simulink model "TCSILOW"  (R2019a)
settings: Solver=VariableStepAuto  StartTime=0.0  StopTime=100  FixedStep=0.001  RelTol=1e-5  AbsTol=1e-5  EnableMultiTasking=on
values from neighbouring files (symbols this model uses):
  beta0 = 47.9602    [Model_Parameter_TCSI_A.m]
  beta2 = 2.1291e-005    (= 2.1291e-05)    [Model_Parameter_TCSI_A.m]
  BSR_opt = 0.9755    [Model_Parameter_TCSI_A.m]
  c_mlin = 1.4021    [Model_Parameter_TCSI_A.m]
  c_mVec = [1.3563 2.7692e+03 0.0100]    [Model_Parameter_TCSI_A.m]
  c_pa = 1011    [Model_Parameter_TCSI_A.m]
  c_pe = 1332    [Model_Parameter_TCSI_A.m]
  c_phi2 = 0    [Model_Parameter_TCSI_A.m]
  c_pi = 0.2708    [Model_Parameter_TCSI_A.m]
  c_psi2 = 0    [Model_Parameter_TCSI_A.m]
  c_wphiVec = [-1.4298e-08 -0.0015 29.6462]    [Model_Parameter_TCSI_A.m]
  c_wpsiVec = [1.0882e-08 -1.7320e-04 1.0286]    [Model_Parameter_TCSI_A.m]
  d_th = 32e-3    (= 0.032)    [Model_Parameter_TCSI_A.m]
  eta0 = 0.41512    [Model_Parameter_TCSI_A.m]
  eta1 = 6.9379e-005    (= 6.9379e-05)    [Model_Parameter_TCSI_A.m]
  eta_cmax = 0.7364    [Model_Parameter_TCSI_A.m]
  eta_tmmax = 0.8180    (= 0.818)    [Model_Parameter_TCSI_A.m]
  gamma0 = 0.5337    [Model_Parameter_TCSI_A.m]
  gamma1 = 4e-3    (= 0.004)    [Model_Parameter_TCSI_A.m]
  gamma2 = -9.4152e-6    (= -9.4152e-06)    [Model_Parameter_TCSI_A.m]
  gamma_a = 1.3964    [Model_Parameter_TCSI_A.m]
  gamma_e = 1.2734    [Model_Parameter_TCSI_A.m]
  I_e = 0.32074    [Model_Parameter_TCSI_A.m]
  J_t = 2.0000e-04    (= 0.0002)    [Model_Parameter_TCSI_A.m]
  kappa = 1.35    [Model_Parameter_TCSI_A.m]
  lambda = 1    [Model_Parameter_TCSI_A.m]
  LHV = 42.5e6    (= 42500000)    [Model_Parameter_TCSI_A.m]
  p_a = 0.98e5    (= 98000)    [Model_Parameter_TCSI_A.m]
  p_e = 1.05e5    (= 105000)    [Model_Parameter_TCSI_A.m]
  p_minit = 3e4    (= 30000)    [Model_Parameter_TCSI_A.m]
  pi_copt = 1.0455    [Model_Parameter_TCSI_A.m]
  Q_c = [3.09189776853185,-2.48232013831700;-2.48232013831700,2.14785596204381]    [Model_Parameter_TCSI_A.m]
  R = 287    [Model_Parameter_TCSI_A.m]
  R_a = 287    [Model_Parameter_TCSI_A.m]
  R_c = 0.0400    (= 0.04)    [Model_Parameter_TCSI_A.m]
  R_t = 0.0400    (= 0.04)    [Model_Parameter_TCSI_A.m]
  sigma_0 = 14.7    [Model_Parameter_TCSI_A.m]
  theta_a = 298    [Model_Parameter_TCSI_A.m]
  theta_exm = 873    [Model_Parameter_TCSI_A.m]
  theta_m = 298    [Model_Parameter_TCSI_A.m]
  u_0 = 0.0039    [Model_Parameter_TCSI_A.m]
  V_c = 1.99e-3    (= 0.00199)    [Model_Parameter_TCSI_A.m]
  V_d = 0.0127    [Model_Parameter_TCSI_A.m]
  V_exm = 0.0012    [Model_Parameter_TCSI_A.m]
  V_m = 16.3210e-3    (= 0.016321)    [Model_Parameter_TCSI_A.m]
  w_copt = 0.2753    [Model_Parameter_TCSI_A.m]
  w_tlin = 2.7969e+03    (= 2796.9)    [Model_Parameter_TCSI_A.m]
undefined symbols (not defined in the file or in its folder): den, num
libraries: simulink x10, cstblocks x1
settings Model: Creator=GOBA  LastModifiedBy=ameya
settings SolverCC: ZeroCrossAlgorithm=Adaptive
settings DataIOCC: ExternalInput=[0 2]  InitialState=[]  LimitDataPoints=on  LoadInitialState=on  SaveFormat=Array  SignalLoggingSaveFormat=ModelDataLogs  ReturnWorkspaceOutputs=off  SignalLoggingName=sigsOut
settings OptimizationCC: DefaultParameterBehavior=Inlined  BufferReuse=off  ExpressionDepthLimit=2147483647  InitFltsAndDblsToZero=on  LifeSpan=inf
settings DebuggingCC: SaveWithParameterizedLinksMsg=none  UnderspecifiedInitializationDetection=Classic  MergeDetectMultiDrivingBlocksExec=none  SignalResolutionControl=TryResolveAllWithWarning  IgnoredZcDiagnostic=none  MultiTaskDSMMsg=warning  MultiTaskCondExecSysMsg=none  FcnCallInpInsideContextMsg=warning  StateNameClashWarn=warning  InitInArrayFormatMsg=none  SFUnexpectedBacktrackingDiag=warning  SFNoUnconditionalDefaultTransitionDiag=warning  SFExecutionAtInitializationDiag=none  ArithmeticOperatorsInVariantConditions=warning
settings HardwareCC: ProdBitPerPointer=32  ProdBitPerSizeT=32  ProdBitPerPtrDiffT=32  ProdLargestAtomicFloat=None  ProdIntDivRoundTo=Undefined  ProdEndianess=Unspecified  ProdWordSize=32  ProdHWDeviceType=32-bit Generic  TargetUnknown=on
settings ModelReferenceCC: PropagateSignalLabelsOutOfModel=off
settings SFSimCC: SimUseLocalCustomCode=off
settings RTWCC: Description=Generic Real-Time Target  RTWUseLocalCustomCode=off
settings CodeAppCC: StateflowObjectComments=on
settings GRTTargetCC: TargetFcnLib=ansi_tfl_tmw.mat  TargetLangStandard=C89/C90 (ANSI)  GeneratePreprocessorConditionals=Disable all  CombineOutputUpdateFcns=off  GRTInterface=on
settings ConfigComp: CovMetricSettings=dw  CovHtmlReporting=on  CovSaveCumulativeToWorkspaceVar=on  CovSaveSingleToWorkspaceVar=on  CovExternalEMLEnable=off

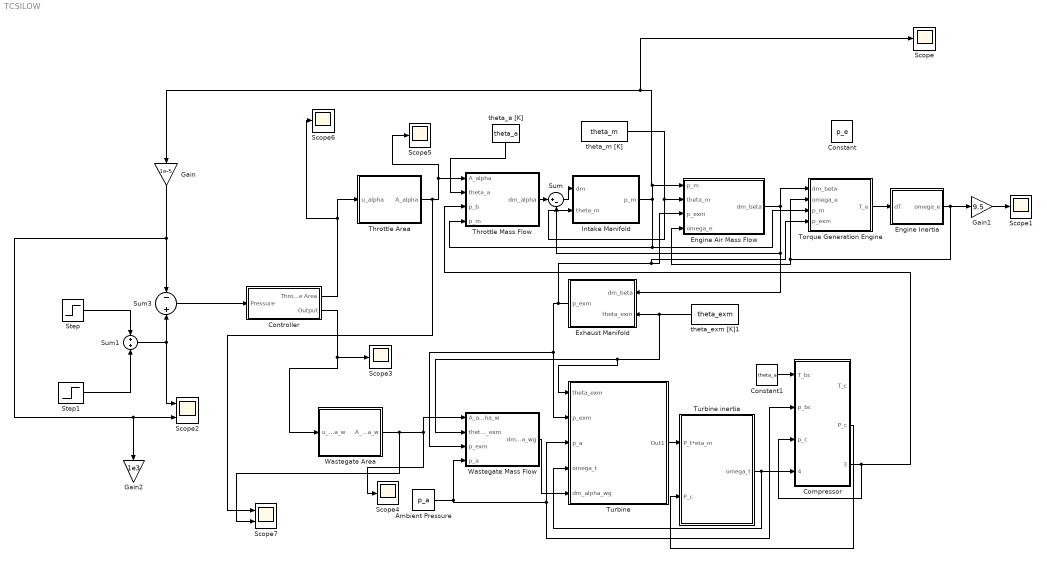
== system TCSILOW ==
  Ambient Pressure : Constant  Value=p_a
  "Compressor " : Subsystem
  Constant : Constant  Value=p_e
  Constant1 : Constant  Value=theta_a
  Controller : Subsystem
  Engine Air Mass Flow : Subsystem
  Engine Inertia : Subsystem
  Exhaust Manifold : Subsystem
  Gain : Gain  Gain=1e-5
  Gain1 : Gain  Gain=9.5
  Gain2 : Gain  Gain=1e3
  Intake Manifold : Subsystem
  Scope{,1,3..6} (6 alike) : Scope
  Scope2 : Scope  NumInputPorts=2
  Scope7 : Scope  NumInputPorts=2
  Step : Step  Time=20  Before=0.3  After=0.6  SampleTime=0
  Step1 : Step  Time=65  After=0.3  SampleTime=0
  Sum : Sum  Inputs=|+-  SaturateOnIntegerOverflow=on
  Sum1 : Sum
  Sum3 : Sum  Inputs=-+
  Throttle Area : Subsystem
  Throttle Mass Flow : Subsystem
  Torque Generation Engine : Subsystem
  "Turbine " : Subsystem
  "Turbine inertia " : Subsystem
  Wastegate Area : Subsystem
  Wastegate Mass Flow : Subsystem
  theta_a [K] : Constant  Value=theta_a
  theta_exm [K]1 : Constant  Value=theta_exm
  theta_m [K] : Constant  Value=theta_m
  wires:
  theta_a [K]/1 -> Throttle Mass Flow/2(theta_a)
  Throttle Mass Flow/1(dm_alpha) -> Sum/1
  Sum/1 -> Intake Manifold/1(dm)
  Torque Generation Engine/1(T_e) -> Engine Inertia/1(dT)
  theta_exm [K]1/1 -> "Turbine "/1(theta_exm), Wastegate Mass Flow/2(theta_exm), Exhaust Manifold/2(theta_exm)
  Exhaust Manifold/1("p_exm ") -> Torque Generation Engine/4(p_exm), Engine Air Mass Flow/3(p_exm), "Turbine "/2(p_exm), Wastegate Mass Flow/3(p_exm)
  Engine Air Mass Flow/1(dm_beta) -> Torque Generation Engine/1(dm_beta), Exhaust Manifold/1(dm_beta), Sum/2
  Wastegate Mass Flow/1(dm_alpha_wg) -> "Turbine "/5(dm_alpha_wg)
  Controller/1(Throttle Area) -> Scope6/1, Throttle Area/1(u_alpha)
  Engine Inertia/1("omega_e ") -> Engine Air Mass Flow/4(omega_e), Torque Generation Engine/2(omega_e), Gain1/1
  Ambient Pressure/1 -> "Compressor "/2(p_bc), "Turbine "/3(p_a), Wastegate Mass Flow/4(p_a)
  Controller/2(Output) -> Scope3/1, Wastegate Area/1(u_alpha_w)
  "Turbine "/1(Out1) -> "Turbine inertia "/1(P_t*eta_m)
  "Turbine inertia "/1(omega_t) -> "Turbine "/4(omega_t), "Compressor "/4(omega_t1)
  "Compressor "/2(P_c) -> "Turbine inertia "/2(P_c)
  "Compressor "/3(p_boost) -> "Compressor "/3(p_c), Throttle Mass Flow/3(p_b)
  Constant1/1 -> "Compressor "/1(T_bc)
  Gain1/1 -> Scope1/1
  Wastegate Area/1(A_alpha_w) -> Scope7/2, Wastegate Mass Flow/1(A_alpha_w), Scope4/1
  Intake Manifold/1("p_m ") -> Torque Generation Engine/3(p_m), Throttle Mass Flow/4(p_m), Engine Air Mass Flow/1(p_m), Scope/1, Gain/1
  Sum3/1 -> Controller/1(Pressure)
  Gain/1 -> Scope2/2, Gain2/1, Sum3/1
  theta_m [K]/1 -> Intake Manifold/2(theta_m), Engine Air Mass Flow/2(theta_m)
  Step/1 -> Sum1/1
  Step1/1 -> Sum1/2
  Sum1/1 -> Sum3/2, Scope2/1
  Throttle Area/1(A_alpha) -> Throttle Mass Flow/1(A_alpha), Scope5/1, Scope7/1

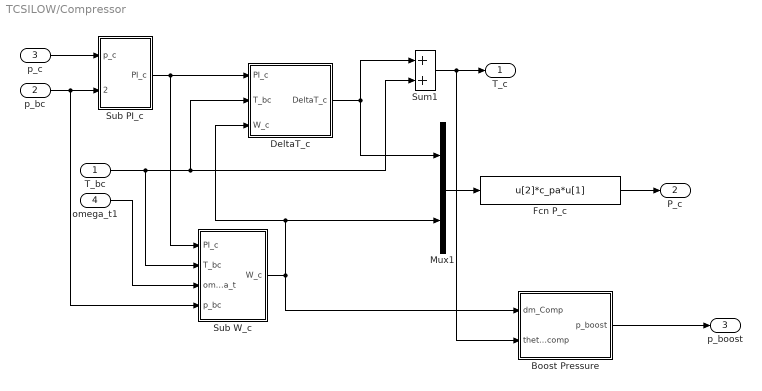
== system TCSILOW/Compressor  ==
  T_bc : Inport
  p_bc : Inport  Port=2
  p_c : Inport  Port=3
  omega_t1 : Inport  Port=4
  Boost Pressure : Subsystem
  DeltaT_c : Subsystem
  Fcn P_c : Fcn  Expr=u[2]*c_pa*u[1]
  Mux1 : Mux  Inputs=2
  Sub PI_c : Subsystem
  Sub W_c : Subsystem
  Sum1 : Sum  SaturateOnIntegerOverflow=on
  T_c : Outport  VectorParamsAs1DForOutWhenUnconnected=on
  P_c : Outport  Port=2  VectorParamsAs1DForOutWhenUnconnected=on
  p_boost : Outport  Port=3
  wires:
  p_bc/1 -> Sub PI_c/2(p_bc), Sub W_c/4(p_bc)
  Sub W_c/1(W_c) -> Boost Pressure/1(dm_Comp), DeltaT_c/3(W_c), Mux1/2
  Sum1/1 -> Boost Pressure/2(theta_comp), T_c/1
  DeltaT_c/1(DeltaT_c) -> Sum1/1, Mux1/1
  Mux1/1 -> Fcn P_c/1
  Sub PI_c/1(PI_c) -> DeltaT_c/1(PI_c), Sub W_c/1(PI_c)
  p_c/1 -> Sub PI_c/1(p_c)
  T_bc/1 -> Sub W_c/2(T_bc), DeltaT_c/2(T_bc), Sum1/2
  omega_t1/1 -> Sub W_c/3(omega_t)
  Fcn P_c/1 -> P_c/1
  Boost Pressure/1("p_boost ") -> p_boost/1

== system TCSILOW/Controller ==
  Pressure : Inport
  Scope : Scope
  Throttle Control : Subsystem
  Wastegate : Subsystem
  Throttle Area : Outport
  Output : Outport  Port=2
  wires:
  Wastegate/1(Output) -> Output/1
  Throttle Control/1(Output) -> Scope/1, Throttle Area/1, Wastegate/1(Throttle Posn)
  Pressure/1 -> Wastegate/2(Pressure), Throttle Control/1(Pressure)

== system TCSILOW/Engine Air Mass Flow ==
  p_m : Inport
  theta_m : Inport  Port=2
  p_exm : Inport  Port=3
  omega_e : Inport  Port=4
  Fcn : Fcn  Expr=u[1]/(R*u[2])*(gamma0+gamma1*u[3]+gamma2*u[3]^2)*((V_c+V_d)/V_d-V_c/V_d*(u[4]/u[1])^(1/kappa))*V_d*u[3]/(4*pi)/(1+1/(lambda*sigma_0))
  Mux1 : Mux
  dm_beta : Outport
  wires:
  Mux1/1 -> Fcn/1
  p_m/1 -> Mux1/1
  theta_m/1 -> Mux1/2
  Fcn/1 -> dm_beta/1
  omega_e/1 -> Mux1/3
  p_exm/1 -> Mux1/4

== system TCSILOW/Engine Inertia ==
  dT : Inport
  Gain : Gain  Gain=1/I_e  SaturateOnIntegerOverflow=on  OutDataTypeStr=Inherit: Same as input  ParamDataTypeStr=Inherit: Same as input
  Saturation : Saturate  UpperLimit=500  LowerLimit=30
  omega_e : Integrator  IgnoreLimit=on
  "omega_e " : Outport
  wires:
  Saturation/1 -> "omega_e "/1
  Gain/1 -> Saturation/1
  dT/1 -> omega_e/1
  omega_e/1 -> Gain/1

== system TCSILOW/Exhaust Manifold ==
  dm_beta : Inport
  theta_exm : Inport  Port=2
  Constant : Constant  Value=R/V_exm
  Product : Product  Inputs=3  SaturateOnIntegerOverflow=on  OutDataTypeStr=Inherit: Same as first input
  p_exm : Integrator  InitialCondition=p_minit
  "p_exm " : Outport
  wires:
  Constant/1 -> Product/1
  Product/1 -> p_exm/1
  dm_beta/1 -> Product/2
  p_exm/1 -> "p_exm "/1
  theta_exm/1 -> Product/3

== system TCSILOW/Intake Manifold ==
  dm : Inport
  theta_m : Inport  Port=2
  Constant : Constant  Value=R/V_m
  Product : Product  Inputs=3  SaturateOnIntegerOverflow=on  OutDataTypeStr=Inherit: Same as first input
  p_m : Integrator  InitialCondition=p_minit
  "p_m " : Outport
  wires:
  Constant/1 -> Product/1
  Product/1 -> p_m/1
  dm/1 -> Product/2
  theta_m/1 -> Product/3
  p_m/1 -> "p_m "/1

== system TCSILOW/Throttle Area ==
  u_alpha : Inport
  Saturation : Saturate  UpperLimit=8*10e-3  LowerLimit=0
  Throttle Area : Fcn  Expr=pi*d_th^2/4*((1-u_0)*u[1]*0.01)
  A_alpha : Outport
  wires:
  u_alpha/1 -> Throttle Area/1
  Throttle Area/1 -> Saturation/1
  Saturation/1 -> A_alpha/1

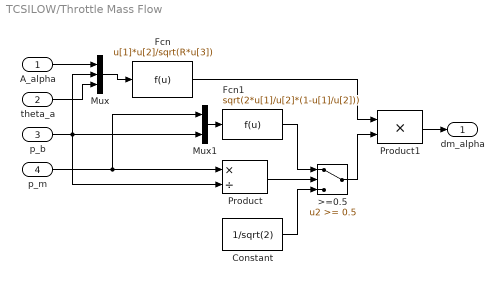
== system TCSILOW/Throttle Mass Flow ==
  A_alpha : Inport
  theta_a : Inport  Port=2
  p_b : Inport  Port=3
  p_m : Inport  Port=4
  >=0.5 : Switch  Threshold=0.5  SaturateOnIntegerOverflow=on
  Constant : Constant  Value=1/sqrt(2)
  Fcn : Fcn  Expr=u[1]*u[2]/sqrt(R*u[3])
  Fcn1 : Fcn  Expr=sqrt(2*u[1]/u[2]*(1-u[1]/u[2]))
  Mux : Mux  Inputs=3
  Mux1 : Mux  Inputs=2
  Product : Product  Inputs=*/  SaturateOnIntegerOverflow=on  OutDataTypeStr=Inherit: Same as first input
  Product1 : Product  SaturateOnIntegerOverflow=on  OutDataTypeStr=Inherit: Same as first input
  dm_alpha : Outport
  wires:
  Mux/1 -> Fcn/1
  p_b/1 -> Mux1/2, Product/2, Mux/2
  Fcn1/1 -> >=0.5/1
  Product/1 -> >=0.5/2
  Constant/1 -> >=0.5/3
  Fcn/1 -> Product1/1
  >=0.5/1 -> Product1/2
  p_m/1 -> Product/1, Mux1/1
  Mux1/1 -> Fcn1/1
  A_alpha/1 -> Mux/1
  theta_a/1 -> Mux/3
  Product1/1 -> dm_alpha/1

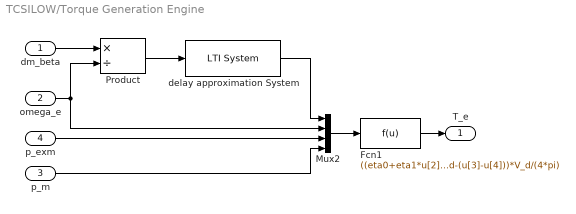
== system TCSILOW/Torque Generation Engine ==
  dm_beta : Inport
  omega_e : Inport  Port=2
  p_m : Inport  Port=3
  p_exm : Inport  Port=4
  Fcn1 : Fcn  Expr=((eta0+eta1*u[2])*LHV*u[1]*4*pi/(lambda*sigma_0*V_d)-(beta0+beta2*u[2]^2)*4*pi/V_d-(u[3]-u[4]))*V_d/(4*pi)
  Mux2 : Mux
  Product : Product  Inputs=*/  SaturateOnIntegerOverflow=on  OutDataTypeStr=Inherit: Same as first input
  delay approximation System : cstblocks/LTI System  sys=tf(num,den)  IC=[]
  T_e : Outport
  wires:
  Mux2/1 -> Fcn1/1
  dm_beta/1 -> Product/1
  omega_e/1 -> Mux2/2, Product/2
  Fcn1/1 -> T_e/1
  p_exm/1 -> Mux2/3
  p_m/1 -> Mux2/4
  Product/1 -> delay approximation System/1
  delay approximation System/1 -> Mux2/1

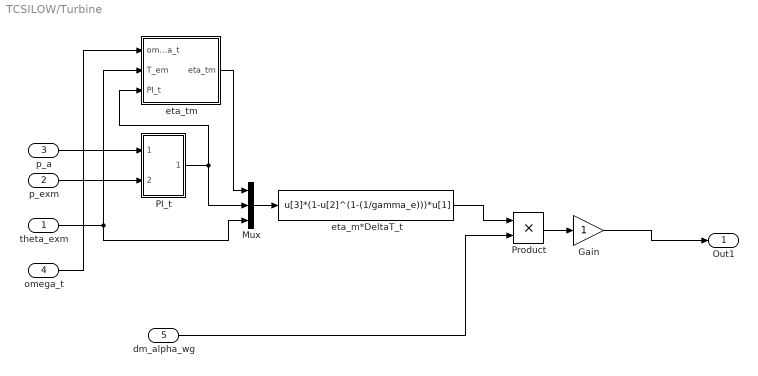
== system TCSILOW/Turbine  ==
  theta_exm : Inport
  p_exm : Inport  Port=2
  p_a : Inport  Port=3
  omega_t : Inport  Port=4
  dm_alpha_wg : Inport  Port=5
  Gain : Gain
  Mux : Mux  Inputs=3
  PI_t : Subsystem
  Product : Product
  eta_m*DeltaT_t : Fcn  Expr=u[3]*(1-u[2]^(1-(1/gamma_e)))*u[1]
  eta_tm : Subsystem
  Out1 : Outport
  wires:
  p_a/1 -> PI_t/1(p_es)
  eta_m*DeltaT_t/1 -> Product/1
  PI_t/1(PI_t) -> eta_tm/3(PI_t), Mux/2
  theta_exm/1 -> Mux/3, eta_tm/2(T_em)
  p_exm/1 -> PI_t/2(p_em)
  Gain/1 -> Out1/1
  Mux/1 -> eta_m*DeltaT_t/1
  eta_tm/1(eta_tm) -> Mux/1
  omega_t/1 -> eta_tm/1(omega_t)
  dm_alpha_wg/1 -> Product/2
  Product/1 -> Gain/1

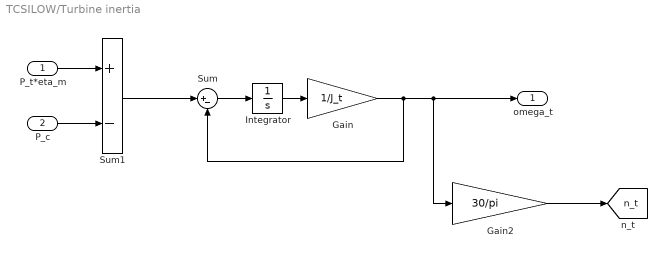
== system TCSILOW/Turbine inertia  ==
  P_t*eta_m : Inport
  P_c : Inport  Port=2
  Gain : Gain  Gain=1/J_t  SaturateOnIntegerOverflow=on  OutDataTypeStr=Inherit: Same as input  ParamDataTypeStr=Inherit: Same as input
  Gain2 : Gain  Gain=30/pi  SaturateOnIntegerOverflow=on  OutDataTypeStr=Inherit: Same as input  ParamDataTypeStr=Inherit: Same as input
  Integrator : Integrator  InitialCondition=0.01  AbsoluteTolerance=0.01
  Sum : Sum  Inputs=|+-
  Sum1 : Sum  Inputs=+-  SaturateOnIntegerOverflow=on
  omega_t : Outport  VectorParamsAs1DForOutWhenUnconnected=on
  tag scope: n_t=global
  wires:
  Integrator/1 -> Gain/1
  P_t*eta_m/1 -> Sum1/1
  Gain2/1 -> [n_t]
  P_c/1 -> Sum1/2
  Sum/1 -> Integrator/1
  Sum1/1 -> Sum/1
  Gain/1 -> Gain2/1, omega_t/1, Sum/2

== system TCSILOW/Wastegate Area ==
  u_alpha_w : Inport
  Saturation : Saturate  UpperLimit=8*10e-3  LowerLimit=0
  Throttle Area : Fcn  Expr=pi*d_th^2/4*(u_0+(1-u_0)*u[1]*0.01)
  A_alpha_w : Outport
  wires:
  u_alpha_w/1 -> Throttle Area/1
  Throttle Area/1 -> Saturation/1
  Saturation/1 -> A_alpha_w/1

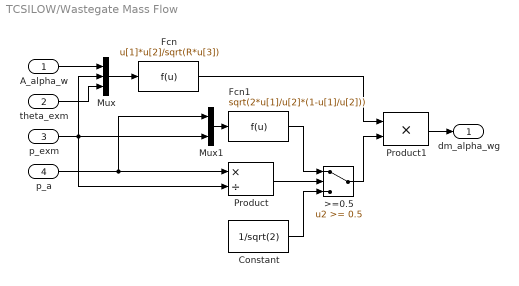
== system TCSILOW/Wastegate Mass Flow ==
  A_alpha_w : Inport
  theta_exm : Inport  Port=2
  p_exm : Inport  Port=3
  p_a : Inport  Port=4
  >=0.5 : Switch  Threshold=0.5  SaturateOnIntegerOverflow=on
  Constant : Constant  Value=1/sqrt(2)
  Fcn : Fcn  Expr=u[1]*u[2]/sqrt(R*u[3])
  Fcn1 : Fcn  Expr=sqrt(2*u[1]/u[2]*(1-u[1]/u[2]))
  Mux : Mux  Inputs=3
  Mux1 : Mux  Inputs=2
  Product : Product  Inputs=*/  SaturateOnIntegerOverflow=on  OutDataTypeStr=Inherit: Same as first input
  Product1 : Product  SaturateOnIntegerOverflow=on  OutDataTypeStr=Inherit: Same as first input
  dm_alpha_wg : Outport
  wires:
  Mux/1 -> Fcn/1
  p_exm/1 -> Mux1/2, Product/2, Mux/2
  Fcn1/1 -> >=0.5/1
  Product/1 -> >=0.5/2
  Constant/1 -> >=0.5/3
  Fcn/1 -> Product1/1
  >=0.5/1 -> Product1/2
  p_a/1 -> Product/1, Mux1/1
  Mux1/1 -> Fcn1/1
  A_alpha_w/1 -> Mux/1
  theta_exm/1 -> Mux/3
  Product1/1 -> dm_alpha_wg/1

== system TCSILOW/Compressor /Boost Pressure ==
  dm_Comp : Inport
  theta_comp : Inport  Port=2
  Constant : Constant  Value=R/V_m
  Product : Product  Inputs=3  SaturateOnIntegerOverflow=on  OutDataTypeStr=Inherit: Same as first input
  p_m : Integrator  InitialCondition=p_minit
  "p_boost " : Outport
  wires:
  Constant/1 -> Product/1
  Product/1 -> p_m/1
  dm_Comp/1 -> Product/2
  p_m/1 -> "p_boost "/1
  theta_comp/1 -> Product/3

== system TCSILOW/Compressor /DeltaT_c ==
  PI_c : Inport
  T_bc : Inport  Port=2
  W_c : Inport  Port=3
  Fcn DeltaT_c : Fcn  Expr=u[3]*(1-u[2]^(1-(1/gamma_a)))*u[1]
  Mux : Mux  Inputs=3
  eta_c : Subsystem
  DeltaT_c : Outport  VectorParamsAs1DForOutWhenUnconnected=on
  wires:
  Fcn DeltaT_c/1 -> DeltaT_c/1
  T_bc/1 -> Mux/3
  PI_c/1 -> Mux/2, eta_c/2(PI_c)
  W_c/1 -> eta_c/1(W_c)
  eta_c/1(eta_c) -> Mux/1
  Mux/1 -> Fcn DeltaT_c/1

== system TCSILOW/Compressor /Sub PI_c ==
  p_c : Inport
  p_bc : Inport  Port=2
  Constant1 : Constant
  Div PI_c : Product  Inputs=*/  SaturateOnIntegerOverflow=on  OutDataTypeStr=Inherit: Same as first input
  MinMax1 : MinMax  Function=max  Inputs=2  SaturateOnIntegerOverflow=on  InputSameDT=on
  PI_c : Outport  VectorParamsAs1DForOutWhenUnconnected=on
  wires:
  MinMax1/1 -> PI_c/1
  p_c/1 -> Div PI_c/1
  p_bc/1 -> Div PI_c/2
  Constant1/1 -> MinMax1/2
  Div PI_c/1 -> MinMax1/1

== system TCSILOW/Compressor /Sub W_c ==
  PI_c : Inport
  T_bc : Inport  Port=2
  omega_t : Inport  Port=3
  p_bc : Inport  Port=4
  Fcn W_c : Fcn  Expr=u[3]*pi*R_c^3*u[1]*u[4]/(R_a*u[2])
  Mux3 : Mux
  PHI_c : Subsystem
  Saturation : Saturate  UpperLimit=inf  LowerLimit=1e-4
  W_c : Outport  VectorParamsAs1DForOutWhenUnconnected=on
  wires:
  Saturation/1 -> W_c/1
  Fcn W_c/1 -> Saturation/1
  PI_c/1 -> PHI_c/1(PI_c)
  p_bc/1 -> Mux3/3
  T_bc/1 -> Mux3/2, PHI_c/2(T_bc)
  omega_t/1 -> Mux3/1, PHI_c/3(omega_t)
  PHI_c/1(PHI_c) -> Mux3/4
  Mux3/1 -> Fcn W_c/1

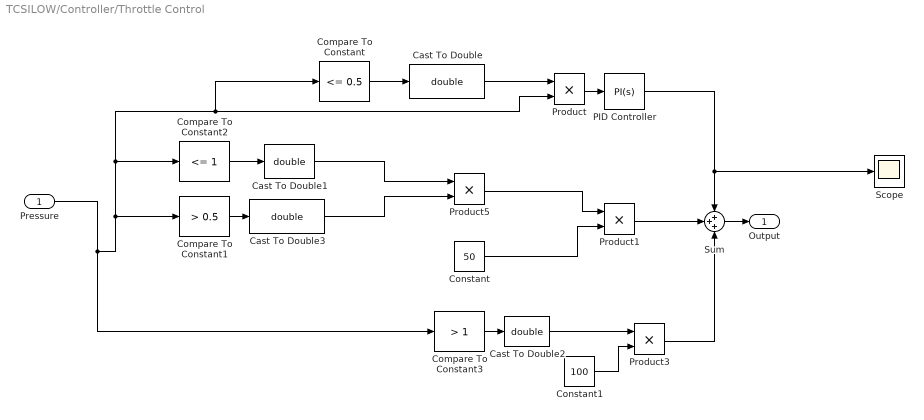
== system TCSILOW/Controller/Throttle Control ==
  Pressure : Inport
  Cast To Double{,1..3} (4 alike) : DataTypeConversion  OutDataTypeStr=double
  Compare To Constant : simulink/Logic and Bit Operations/Compare To Constant  relop=<=  const=0.5  OutDataTypeStr=boolean
  Compare To Constant1 : simulink/Logic and Bit Operations/Compare To Constant  relop=>  const=0.5  OutDataTypeStr=boolean
  Compare To Constant2 : simulink/Logic and Bit Operations/Compare To Constant  relop=<=  const=1  OutDataTypeStr=boolean
  Compare To Constant3 : simulink/Logic and Bit Operations/Compare To Constant  relop=>  const=1  OutDataTypeStr=boolean
  Constant : Constant  Value=50
  Constant1 : Constant  Value=100
  PID Controller : simulink/Continuous/PID Controller  Controller=PI  Form=Parallel  TimeDomain=Continuous-time  SampleTime=-1  IntegratorMethod=Forward Euler  FilterMethod=Forward Euler  ControllerParametersSource=internal  P=50  I=75  D=-1.56475599559011  UseFilter=on  N=1.4222540202283  TunerSelectOption=Transfer Function Based (PID Tuner App)  InitialConditionSource=internal  InitialConditionForIntegrator=0  InitialConditionForFilter=0  DifferentiatorICPrevScaledInput=0  ExternalReset=none  TrackingMode=off  Kt=1  LimitOutput=off  UpperSaturationLimit=inf  LowerSaturationLimit=-inf  LinearizeAsGain=on  AntiWindupMode=none  Kb=1  POutMin=[]  POutMax=[]  IOutMin=[]  IOutMax=[]  DOutMin=[]  DOutMax=[]  NOutMin=[]  NOutMax=[]  SumOutMin=[]  SumOutMax=[]  SaturationOutMin=[]  SaturationOutMax=[]  PParamMin=[]  PParamMax=[]  IParamMin=[]  IParamMax=[]  DParamMin=[]  DParamMax=[]  NParamMin=[]  NParamMax=[]  KbParamMin=[]  KbParamMax=[]  KtParamMin=[]  KtParamMax=[]  KbOutMin=[]  KbOutMax=[]  KtOutMin=[]  KtOutMax=[]  IntegratorOutMin=[]  IntegratorOutMax=[]  FilterOutMin=[]  FilterOutMax=[]  SumI1OutMin=[]  SumI1OutMax=[]  SumI2OutMin=[]  SumI2OutMax=[]  SumI3OutMin=[]  SumI3OutMax=[]  SumI4OutMin=[]  SumI4OutMax=[]  SumDOutMin=[]  SumDOutMax=[]  DifferentiatorOutMin=[]  DifferentiatorOutMax=[]  FilterDiffOutCoefMin=[]  FilterDiffOutCoefMax=[]  ReciprocalOutMin=[]  ReciprocalOutMax=[]  SumDenOutMin=[]  SumDenOutMax=[]  SumNumOutMin=[]  SumNumOutMax=[]  DivideOutMin=[]  DivideOutMax=[]  IntegratorContinuousStateAttributes=''  IntegratorStateMustResolveToSignalObject=off  IntegratorRTWStateStorageClass=Auto  FilterContinuousStateAttributes=''  FilterStateMustResolveToSignalObject=off  FilterRTWStateStorageClass=Auto  ParallelPVariant=InternalParameters  IdealPVariant=Disabled  IVariant=InternalParameters  DVariant=Disabled  IntegratorVariant=Continuous  SatVariant=Disabled  AWVariant=Passthrough  PCopyVariant=Disabled  TRVariant=Disabled  FdbkBlocksVariant=Forward  IdealPFdbkVariant=Disabled  SatFdbkVariant=Disabled  DerivativeFilterVariant=Disabled  NVariant=Disabled  NCopyVariant=Disabled_SignalSpec  FilterICVariant=Disabled  IntegratorICVariant=InternalICs  ExternalResetVariant=Disabled  TRSumVariant=Passthrough  SumFdbkVariant=Disabled  SumVariant=Sum_PI
  Product{,1,3,5} (4 alike) : Product
  Scope : Scope
  Sum : Sum  Inputs=+++
  Output : Outport
  wires:
  Compare To Constant/1 -> Cast To Double/1
  Constant/1 -> Product1/2
  Compare To Constant3/1 -> Cast To Double2/1
  Product/1 -> PID Controller/1
  Product3/1 -> Sum/3
  Cast To Double2/1 -> Product3/1
  Constant1/1 -> Product3/2
  Cast To Double/1 -> Product/1
  Cast To Double1/1 -> Product5/1
  Sum/1 -> Output/1
  Compare To Constant1/1 -> Cast To Double3/1
  Cast To Double3/1 -> Product5/2
  Compare To Constant2/1 -> Cast To Double1/1
  Product5/1 -> Product1/1
  Product1/1 -> Sum/2
  Pressure/1 -> Compare To Constant3/1, Compare To Constant/1, Product/2, Compare To Constant2/1, Compare To Constant1/1
  PID Controller/1 -> Scope/1, Sum/1

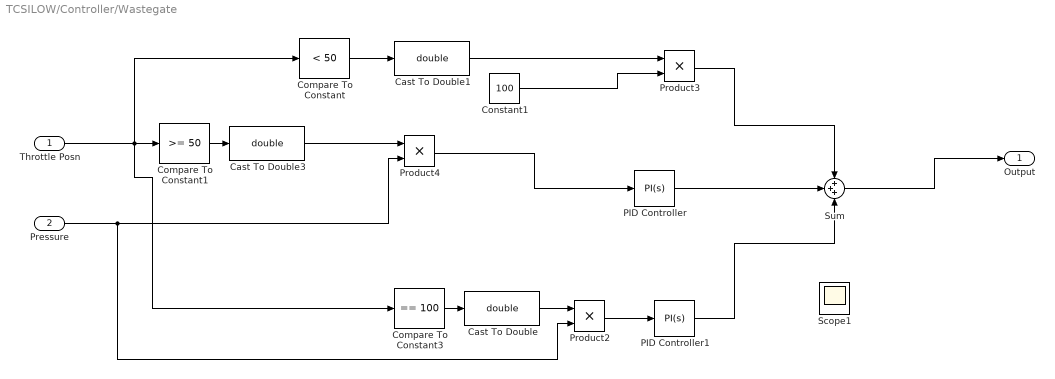
== system TCSILOW/Controller/Wastegate ==
  Throttle Posn : Inport
  Pressure : Inport  Port=2
  Cast To Double : DataTypeConversion  OutDataTypeStr=double
  Cast To Double1 : DataTypeConversion  OutDataTypeStr=double
  Cast To Double3 : DataTypeConversion  OutDataTypeStr=double
  Compare To Constant : simulink/Logic and Bit Operations/Compare To Constant  relop=<  const=50  OutDataTypeStr=boolean
  Compare To Constant1 : simulink/Logic and Bit Operations/Compare To Constant  relop=>=  const=50  OutDataTypeStr=boolean
  Compare To Constant3 : simulink/Logic and Bit Operations/Compare To Constant  relop===  const=100  OutDataTypeStr=boolean
  Constant1 : Constant  Value=100
  PID Controller : simulink/Continuous/PID Controller  Controller=PI  Form=Parallel  TimeDomain=Continuous-time  SampleTime=-1  IntegratorMethod=Forward Euler  FilterMethod=Forward Euler  ControllerParametersSource=internal  P=20  I=50  D=0  UseFilter=on  N=100  TunerSelectOption=Transfer Function Based (PID Tuner App)  InitialConditionSource=internal  InitialConditionForIntegrator=0  InitialConditionForFilter=0  DifferentiatorICPrevScaledInput=0  ExternalReset=none  TrackingMode=off  Kt=1  LimitOutput=off  UpperSaturationLimit=inf  LowerSaturationLimit=-inf  LinearizeAsGain=on  AntiWindupMode=none  Kb=1  POutMin=[]  POutMax=[]  IOutMin=[]  IOutMax=[]  DOutMin=[]  DOutMax=[]  NOutMin=[]  NOutMax=[]  SumOutMin=[]  SumOutMax=[]  SaturationOutMin=[]  SaturationOutMax=[]  PParamMin=[]  PParamMax=[]  IParamMin=[]  IParamMax=[]  DParamMin=[]  DParamMax=[]  NParamMin=[]  NParamMax=[]  KbParamMin=[]  KbParamMax=[]  KtParamMin=[]  KtParamMax=[]  KbOutMin=[]  KbOutMax=[]  KtOutMin=[]  KtOutMax=[]  IntegratorOutMin=[]  IntegratorOutMax=[]  FilterOutMin=[]  FilterOutMax=[]  SumI1OutMin=[]  SumI1OutMax=[]  SumI2OutMin=[]  SumI2OutMax=[]  SumI3OutMin=[]  SumI3OutMax=[]  SumI4OutMin=[]  SumI4OutMax=[]  SumDOutMin=[]  SumDOutMax=[]  DifferentiatorOutMin=[]  DifferentiatorOutMax=[]  FilterDiffOutCoefMin=[]  FilterDiffOutCoefMax=[]  ReciprocalOutMin=[]  ReciprocalOutMax=[]  SumDenOutMin=[]  SumDenOutMax=[]  SumNumOutMin=[]  SumNumOutMax=[]  DivideOutMin=[]  DivideOutMax=[]  IntegratorContinuousStateAttributes=''  IntegratorStateMustResolveToSignalObject=off  IntegratorRTWStateStorageClass=Auto  FilterContinuousStateAttributes=''  FilterStateMustResolveToSignalObject=off  FilterRTWStateStorageClass=Auto  ParallelPVariant=InternalParameters  IdealPVariant=Disabled  IVariant=InternalParameters  DVariant=Disabled  IntegratorVariant=Continuous  SatVariant=Disabled  AWVariant=Passthrough  PCopyVariant=Disabled  TRVariant=Disabled  FdbkBlocksVariant=Forward  IdealPFdbkVariant=Disabled  SatFdbkVariant=Disabled  DerivativeFilterVariant=Disabled  NVariant=Disabled  NCopyVariant=Disabled_SignalSpec  FilterICVariant=Disabled  IntegratorICVariant=InternalICs  ExternalResetVariant=Disabled  TRSumVariant=Passthrough  SumFdbkVariant=Disabled  SumVariant=Sum_PI
  PID Controller1 : simulink/Continuous/PID Controller  Controller=PI  Form=Parallel  TimeDomain=Continuous-time  SampleTime=-1  IntegratorMethod=Forward Euler  FilterMethod=Forward Euler  ControllerParametersSource=internal  P=0  I=-1  D=0  UseFilter=on  N=100  TunerSelectOption=Transfer Function Based (PID Tuner App)  InitialConditionSource=internal  InitialConditionForIntegrator=0  InitialConditionForFilter=0  DifferentiatorICPrevScaledInput=0  ExternalReset=none  TrackingMode=off  Kt=1  LimitOutput=off  UpperSaturationLimit=inf  LowerSaturationLimit=-inf  LinearizeAsGain=on  AntiWindupMode=none  Kb=1  POutMin=[]  POutMax=[]  IOutMin=[]  IOutMax=[]  DOutMin=[]  DOutMax=[]  NOutMin=[]  NOutMax=[]  SumOutMin=[]  SumOutMax=[]  SaturationOutMin=[]  SaturationOutMax=[]  PParamMin=[]  PParamMax=[]  IParamMin=[]  IParamMax=[]  DParamMin=[]  DParamMax=[]  NParamMin=[]  NParamMax=[]  KbParamMin=[]  KbParamMax=[]  KtParamMin=[]  KtParamMax=[]  KbOutMin=[]  KbOutMax=[]  KtOutMin=[]  KtOutMax=[]  IntegratorOutMin=[]  IntegratorOutMax=[]  FilterOutMin=[]  FilterOutMax=[]  SumI1OutMin=[]  SumI1OutMax=[]  SumI2OutMin=[]  SumI2OutMax=[]  SumI3OutMin=[]  SumI3OutMax=[]  SumI4OutMin=[]  SumI4OutMax=[]  SumDOutMin=[]  SumDOutMax=[]  DifferentiatorOutMin=[]  DifferentiatorOutMax=[]  FilterDiffOutCoefMin=[]  FilterDiffOutCoefMax=[]  ReciprocalOutMin=[]  ReciprocalOutMax=[]  SumDenOutMin=[]  SumDenOutMax=[]  SumNumOutMin=[]  SumNumOutMax=[]  DivideOutMin=[]  DivideOutMax=[]  IntegratorContinuousStateAttributes=''  IntegratorStateMustResolveToSignalObject=off  IntegratorRTWStateStorageClass=Auto  FilterContinuousStateAttributes=''  FilterStateMustResolveToSignalObject=off  FilterRTWStateStorageClass=Auto  ParallelPVariant=InternalParameters  IdealPVariant=Disabled  IVariant=InternalParameters  DVariant=Disabled  IntegratorVariant=Continuous  SatVariant=Disabled  AWVariant=Passthrough  PCopyVariant=Disabled  TRVariant=Disabled  FdbkBlocksVariant=Forward  IdealPFdbkVariant=Disabled  SatFdbkVariant=Disabled  DerivativeFilterVariant=Disabled  NVariant=Disabled  NCopyVariant=Disabled_SignalSpec  FilterICVariant=Disabled  IntegratorICVariant=InternalICs  ExternalResetVariant=Disabled  TRSumVariant=Passthrough  SumFdbkVariant=Disabled  SumVariant=Sum_PI
  Product2 : Product
  Product3 : Product
  Product4 : Product
  Scope1 : Scope
  Sum : Sum  Inputs=+++
  Output : Outport
  wires:
  Sum/1 -> Output/1
  PID Controller/1 -> Sum/2
  Throttle Posn/1 -> Compare To Constant3/1, Compare To Constant/1, Compare To Constant1/1
  Cast To Double1/1 -> Product3/1
  Compare To Constant3/1 -> Cast To Double/1
  Compare To Constant/1 -> Cast To Double1/1
  Constant1/1 -> Product3/2
  Product2/1 -> PID Controller1/1
  PID Controller1/1 -> Sum/3
  Cast To Double/1 -> Product2/1
  Compare To Constant1/1 -> Cast To Double3/1
  Product3/1 -> Sum/1
  Cast To Double3/1 -> Product4/1
  Product4/1 -> PID Controller/1
  Pressure/1 -> Product2/2, Product4/2

== system TCSILOW/Turbine /PI_t ==
  p_es : Inport
  p_em : Inport  Port=2
  Constant : Constant  Value=0.9999
  Div PI_t : Product  Inputs=*/  SaturateOnIntegerOverflow=on  OutDataTypeStr=Inherit: Same as first input
  MinMax : MinMax  Inputs=2  SaturateOnIntegerOverflow=on  InputSameDT=on
  PI_t : Outport  VectorParamsAs1DForOutWhenUnconnected=on
  wires:
  MinMax/1 -> PI_t/1
  p_es/1 -> Div PI_t/1
  p_em/1 -> Div PI_t/2
  Div PI_t/1 -> MinMax/1
  Constant/1 -> MinMax/2

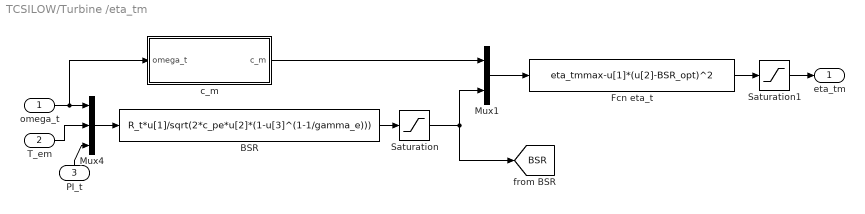
== system TCSILOW/Turbine /eta_tm ==
  omega_t : Inport
  T_em : Inport  Port=2
  PI_t : Inport  Port=3
  BSR : Fcn  Expr=R_t*u[1]/sqrt(2*c_pe*u[2]*(1-u[3]^(1-1/gamma_e)))
  Fcn eta_t : Fcn  Expr=eta_tmmax-u[1]*(u[2]-BSR_opt)^2
  Mux1 : Mux  Inputs=2
  Mux4 : Mux  Inputs=3
  Saturation : Saturate  UpperLimit=2*BSR_opt  LowerLimit=0
  Saturation1 : Saturate  UpperLimit=1  LowerLimit=0.2
  c_m : Subsystem
  eta_tm : Outport  VectorParamsAs1DForOutWhenUnconnected=on
  tag scope: BSR=global
  wires:
  c_m/1(c_m) -> Mux1/1
  Saturation/1 -> [BSR], Mux1/2
  Mux1/1 -> Fcn eta_t/1
  Saturation1/1 -> eta_tm/1
  Fcn eta_t/1 -> Saturation1/1
  PI_t/1 -> Mux4/3
  T_em/1 -> Mux4/2
  omega_t/1 -> c_m/1(omega_t), Mux4/1
  BSR/1 -> Saturation/1
  Mux4/1 -> BSR/1

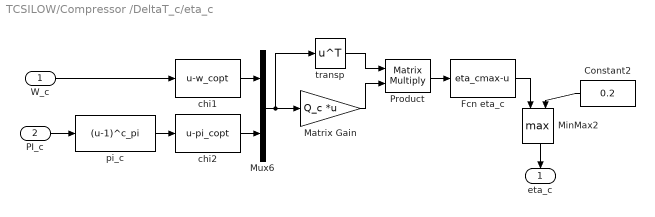
== system TCSILOW/Compressor /DeltaT_c/eta_c ==
  W_c : Inport
  PI_c : Inport  Port=2
  Constant2 : Constant  Value=0.2
  Fcn eta_c : Fcn  Expr=eta_cmax-u
  Matrix Gain : Gain  Gain=Q_c  Multiplication=Matrix(K*u)  SaturateOnIntegerOverflow=on  OutDataTypeStr=Inherit: Same as input  ParamDataTypeStr=Inherit: Same as input
  MinMax2 : MinMax  Function=max  Inputs=2  SaturateOnIntegerOverflow=on  InputSameDT=on
  Mux6 : Mux  Inputs=2
  Product : Product  Multiplication=Matrix(*)  SaturateOnIntegerOverflow=on  OutDataTypeStr=Inherit: Same as first input
  chi1 : Fcn  Expr=u-w_copt
  chi2 : Fcn  Expr=u-pi_copt
  pi_c : Fcn  Expr=(u-1)^c_pi
  transp : Math  Operator=transpose  SaturateOnIntegerOverflow=on
  eta_c : Outport  VectorParamsAs1DForOutWhenUnconnected=on
  wires:
  W_c/1 -> chi1/1
  MinMax2/1 -> eta_c/1
  PI_c/1 -> pi_c/1
  Constant2/1 -> MinMax2/2
  Fcn eta_c/1 -> MinMax2/1
  Product/1 -> Fcn eta_c/1
  Matrix Gain/1 -> Product/2
  transp/1 -> Product/1
  Mux6/1 -> transp/1, Matrix Gain/1
  chi2/1 -> Mux6/2
  chi1/1 -> Mux6/1
  pi_c/1 -> chi2/1

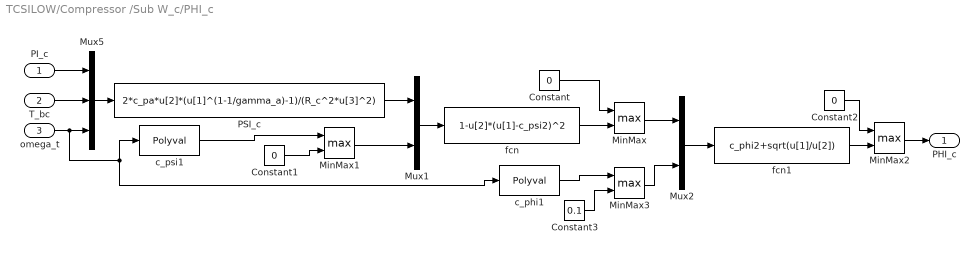
== system TCSILOW/Compressor /Sub W_c/PHI_c ==
  PI_c : Inport
  T_bc : Inport  Port=2
  omega_t : Inport  Port=3
  Constant : Constant  Value=0
  Constant1 : Constant  Value=0
  Constant2 : Constant  Value=0
  Constant3 : Constant  Value=0.1
  MinMax{,1..3} (4 alike) : MinMax  Function=max  Inputs=2  SaturateOnIntegerOverflow=on  InputSameDT=on
  Mux1 : Mux  Inputs=2
  Mux2 : Mux  Inputs=2
  Mux5 : Mux  Inputs=3
  PSI_c : Fcn  Expr=2*c_pa*u[2]*(u[1]^(1-1/gamma_a)-1)/(R_c^2*u[3]^2)
  c_phi1 : Polyval  Coefs=c_wphiVec
  c_psi1 : Polyval  Coefs=c_wpsiVec
  fcn : Fcn  Expr=1-u[2]*(u[1]-c_psi2)^2
  fcn1 : Fcn  Expr=c_phi2+sqrt(u[1]/u[2])
  PHI_c : Outport  VectorParamsAs1DForOutWhenUnconnected=on
  wires:
  Constant3/1 -> MinMax3/2
  MinMax3/1 -> Mux2/2
  c_phi1/1 -> MinMax3/1
  MinMax2/1 -> PHI_c/1
  fcn1/1 -> MinMax2/2
  Constant2/1 -> MinMax2/1
  Mux2/1 -> fcn1/1
  MinMax/1 -> Mux2/1
  fcn/1 -> MinMax/2
  Constant/1 -> MinMax/1
  MinMax1/1 -> Mux1/2
  c_psi1/1 -> MinMax1/1
  Constant1/1 -> MinMax1/2
  Mux1/1 -> fcn/1
  PSI_c/1 -> Mux1/1
  omega_t/1 -> c_phi1/1, c_psi1/1, Mux5/3
  T_bc/1 -> Mux5/2
  PI_c/1 -> Mux5/1
  Mux5/1 -> PSI_c/1

== system TCSILOW/Turbine /eta_tm/c_m ==
  omega_t : Inport
  Constant : Constant  Value=c_mVec(2)
  MinMax : MinMax  Function=max  Inputs=2  SaturateOnIntegerOverflow=on  InputSameDT=on
  Switch PSI : Switch  Threshold=w_tlin  SaturateOnIntegerOverflow=on
  c_m linear : Fcn  Expr=c_mlin*(u-c_mVec(2))/(w_tlin-c_mVec(2))
  c_m power : Fcn  Expr=c_mVec(1)*(u-c_mVec(2))^c_mVec(3)
  c_m : Outport  VectorParamsAs1DForOutWhenUnconnected=on
  wires:
  Switch PSI/1 -> c_m/1
  c_m linear/1 -> Switch PSI/3
  c_m power/1 -> Switch PSI/1
  omega_t/1 -> MinMax/2
  Constant/1 -> MinMax/1
  MinMax/1 -> c_m linear/1, Switch PSI/2, c_m power/1
